simulink library "FSW_Lib"  (R2018b)
settings: Solver=VariableStepAuto  StartTime=0.0  StopTime=10.0  RelTol=1e-3
libraries: actuator_processing_lib x1, allocation_lib x1, control_command_generation_lib x1, evironmentEstimation_lib x1, mode_select_lib x1, target_gen_lib_nadir x1
settings Model: Creator=colem  LastModifiedBy=colem

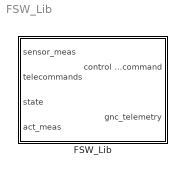
== system FSW_Lib ==
  FSW_Lib : Subsystem

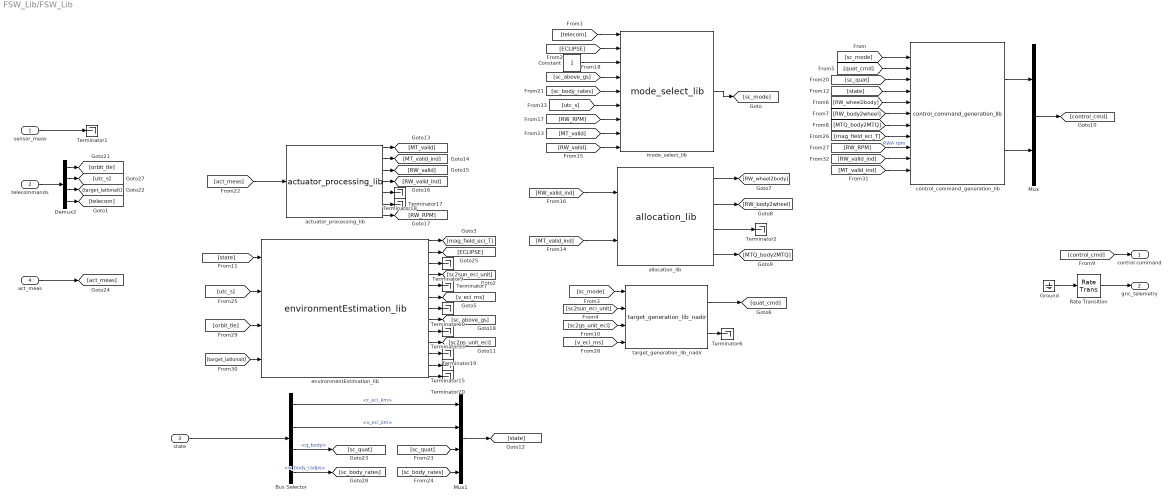
== system FSW_Lib/FSW_Lib ==
  sensor_meas : Inport
  telecommands : Inport  Port=2
  state : Inport  Port=3
  act_meas : Inport  Port=4
  Bus Selector : BusSelector  OutputSignals=r_eci_km,v_eci_km,q_body,w_body_radps
  Constant : Constant
  Demux2 : Demux  Outputs=[9 1 3 7]
  Ground : Ground
  Mux : Mux  Inputs=[4 5]
  Mux1 : Mux  Inputs=[3 3 4 3]
  Rate Transition : RateTransition  OutPortSampleTime=fswParams.sample_time_s
  Terminator{1..2,6..7,9..10,13,15,17..20} (12 alike) : Terminator
  actuator_processing_lib : actuator_processing_lib/actuator_processing_lib  SystemSampleTime=-1
  allocation_lib : allocation_lib/allocation_lib  SystemSampleTime=-1
  control_command_generation_lib : control_command_generation_lib/control_command_generation_lib  SystemSampleTime=-1
  environmentEstimation_lib : evironmentEstimation_lib/environmentEstimation_lib  SystemSampleTime=-1
  mode_select_lib : mode_select_lib/mode_select_lib  SystemSampleTime=-1
  target_generation_lib_nadir : target_gen_lib_nadir/target_generation_lib_nadir  SystemSampleTime=-1
  control command : Outport
  gnc_telemetry : Outport  Port=2
  wires:
  Mux1/1 -> [state]
  [sc_body_rates] -> Mux1/4
  [sc_quat] -> Mux1/3
  Bus Selector/1 -> Mux1/1  "<r_eci_km>"
  Bus Selector/4 -> [sc_body_rates]  "<w_body_radps>"
  Bus Selector/2 -> Mux1/2  "<v_eci_km>"
  Bus Selector/3 -> [sc_quat]  "<q_body>"
  sensor_meas/1 -> Terminator1/1
  telecommands/1 -> Demux2/1
  Ground/1 -> Rate Transition/1
  [control_cmd] -> control command/1
  mode_select_lib/1 -> [sc_mode]
  [sc_mode] -> control_command_generation_lib/1
  [telecom] -> mode_select_lib/1
  [ECLIPSE] -> mode_select_lib/2
  [sc_above_gs] -> mode_select_lib/4
  [sc_body_rates] -> mode_select_lib/5
  [RW_RPM] -> mode_select_lib/7
  Constant/1 -> mode_select_lib/3
  [MT_valid] -> mode_select_lib/8
  [RW_valid] -> mode_select_lib/9
  [sc_mode] -> target_generation_lib_nadir/1
  [sc2sun_eci_unit] -> target_generation_lib_nadir/2
  target_generation_lib_nadir/2 -> Terminator6/1
  [quat_cmd] -> control_command_generation_lib/2
  [RW_valid_ind] -> allocation_lib/1
  [MT_valid_ind] -> allocation_lib/2
  [sc_quat] -> control_command_generation_lib/3
  allocation_lib/1 -> [RW_wheel2body]
  allocation_lib/2 -> [RW_body2wheel]
  [RW_wheel2body] -> control_command_generation_lib/5
  allocation_lib/3 -> Terminator2/1
  allocation_lib/4 -> [MTQ_body2MTQ]
  [RW_body2wheel] -> control_command_generation_lib/6
  [MTQ_body2MTQ] -> control_command_generation_lib/7
  control_command_generation_lib/2 -> Mux/2
  control_command_generation_lib/1 -> Mux/1
  Mux/1 -> [control_cmd]
  environmentEstimation_lib/1 -> [mag_field_eci_T]
  environmentEstimation_lib/2 -> [ECLIPSE]
  environmentEstimation_lib/3 -> Terminator9/1
  environmentEstimation_lib/4 -> [sc2sun_eci_unit]
  environmentEstimation_lib/5 -> Terminator7/1
  environmentEstimation_lib/6 -> [v_eci_ms]
  environmentEstimation_lib/7 -> Terminator10/1
  environmentEstimation_lib/8 -> [sc_above_gs]
  environmentEstimation_lib/9 -> Terminator13/1
  environmentEstimation_lib/10 -> [sc2gs_unit_eci]
  [utc_s] -> environmentEstimation_lib/2
  [orbit_tle] -> environmentEstimation_lib/3
  [sc2gs_unit_eci] -> target_generation_lib_nadir/3
  state/1 -> Bus Selector/1
  [state] -> environmentEstimation_lib/1
  [state] -> control_command_generation_lib/4
  act_meas/1 -> [act_meas]
  actuator_processing_lib/1 -> [MT_valid]
  actuator_processing_lib/2 -> [MT_valid_ind]
  actuator_processing_lib/3 -> [RW_valid]
  actuator_processing_lib/4 -> [RW_valid_ind]
  actuator_processing_lib/5 -> Terminator18/1
  actuator_processing_lib/6 -> Terminator17/1
  actuator_processing_lib/7 -> [RW_RPM]
  [act_meas] -> actuator_processing_lib/1
  environmentEstimation_lib/12 -> Terminator15/1
  environmentEstimation_lib/13 -> Terminator20/1
  environmentEstimation_lib/11 -> Terminator19/1
  Demux2/4 -> [telecom]
  Demux2/2 -> [utc_s]
  [mag_field_eci_T] -> control_command_generation_lib/8
  [RW_RPM] -> control_command_generation_lib/9  "RWA rpm"
  [v_eci_ms] -> target_generation_lib_nadir/4
  Demux2/1 -> [orbit_tle]
  Demux2/3 -> [target_latlonalt]
  [target_latlonalt] -> environmentEstimation_lib/4
  target_generation_lib_nadir/1 -> [quat_cmd]
  Rate Transition/1 -> gnc_telemetry/1
  [RW_valid_ind] -> control_command_generation_lib/10
  [MT_valid_ind] -> control_command_generation_lib/11
  [utc_s] -> mode_select_lib/6
